simulink model "Katex_FullCar_R2017b_V03"  (R2026a)
settings: Solver=ode1  StopTime=1000  FixedStep=Ts  EnableMultiTasking=on
PostLoadFcn:
  | , if any(exist('dsrtsu_mdlpostloadfcn', 'file') == [2, 3, 6]), try dsrtsu_mdlpostloadfcn('Execute', bdroot); catch fprintf('Error in PostLoadFcn (dsrtsu_mdlpostloadfcn) for model "%s":\n %s\n', bdroot, lasterr); end, end,
  | , if any(exist('dsrtsu_mdlpostloadfcn', 'file') ~= 0), dsrtsu_mdlpostloadfcn('Execute', bdroot); end,
InitFcn:
  | , if any(exist('rtifpga_mdlclblib', 'file') ~= 0), rtifpga_mdlclblib('Init', bdroot); end,
  | 
  | 
  | init
undefined symbols (not defined in the file): locklim_sus, roundN, Ts
libraries: sl_discontinuities x29, simulink_extras x26, simulink x22, mjLib x1
(part 4 of 10)

== system Katex_FullCar_R2017b_V03/MuJoCo Interface/RR_Motor_Control/Drv_Driver ==
  In1 : Inport
  In2 : Inport  Port=2
  If1 : If  IfExpression=u1 == 0  ElseIfExpressions=u1 == 1,u1 == 2
  Merge : Merge  Inputs=3
  Position Mode : Subsystem  TreatAsAtomicUnit=on
  Torque Mode : Subsystem  TreatAsAtomicUnit=on
  Velocity Mode : Subsystem  TreatAsAtomicUnit=on
  RR_drive_motor : Outport
  wires:
  [wheel_radius] -> Velocity Mode/5(In5)
  [RRdrv_angvel_rads] -> Velocity Mode/4(In4)
  [drv_motor_freq] -> Velocity Mode/3(In3)
  [drv_motor_zeta] -> Velocity Mode/2(In2)
  Merge/1 -> RR_drive_motor/1
  In2/1 -> Position Mode/1(In1), Velocity Mode/1(In1), Torque Mode/1(In1)
  Velocity Mode/1(controlgain) -> Merge/2
  In1/1 -> If1/1
  Torque Mode/1(controlgain) -> Merge/3
  Position Mode/1(Out1) -> Merge/1
  If1/3 -> Torque Mode/Action
  If1/2 -> Velocity Mode/Action
  If1/1 -> Position Mode/Action

== system Katex_FullCar_R2017b_V03/MuJoCo Interface/RR_Motor_Control/Str_Driver ==
  In1 : Inport
  In2 : Inport  Port=2
  If1 : If  IfExpression=u1 == 0  ElseIfExpressions=u1 == 1,u1 == 2
  Merge : Merge  Inputs=3
  Position Mode : Subsystem  TreatAsAtomicUnit=on
  Torque Mode : Subsystem  TreatAsAtomicUnit=on
  Velocity Mode : Subsystem  TreatAsAtomicUnit=on
  RR_steer_motor : Outport
  wires:
  [RRstr_angvel_rads] -> Position Mode/5(velocity_rad_s)
  [RRstr_ang_rad] -> Position Mode/4(In4)
  [str_motor_freq] -> Position Mode/3(In3)
  [str_motor_zeta] -> Position Mode/2(In2)
  If1/1 -> Position Mode/Action
  If1/2 -> Velocity Mode/Action
  If1/3 -> Torque Mode/Action
  Position Mode/1(Out1) -> Merge/1
  Torque Mode/1(controlgain) -> Merge/3
  In1/1 -> If1/1
  Velocity Mode/1(Out1) -> Merge/2
  In2/1 -> Torque Mode/1(In1), Velocity Mode/1(In1), Position Mode/1(In1)
  Merge/1 -> RR_steer_motor/1

== system Katex_FullCar_R2017b_V03/MuJoCo Interface/RR_Motor_Control/Sus_Driver ==
  In1 : Inport
  In2 : Inport  Port=2
  If1 : If  IfExpression=u1 == 0  ElseIfExpressions=u1 == 1,u1 == 2
  Merge : Merge  Inputs=3
  Position Mode : Subsystem  TreatAsAtomicUnit=on
  Torque Mode : Subsystem  TreatAsAtomicUnit=on
  Velocity Mode : Subsystem  TreatAsAtomicUnit=on
  RR_sus_motor : Outport
  wires:
  [RRsus_angvel_rads] -> Position Mode/5(velocity_rad_s)
  [RRsus_ang_rad] -> Position Mode/4(In4)
  [sus_motor_freq] -> Position Mode/3(In3)
  [sus_motor_zeta] -> Position Mode/2(In2)
  Merge/1 -> RR_sus_motor/1
  In2/1 -> Velocity Mode/1(In1), Torque Mode/1(In1), Position Mode/1(In1)
  Velocity Mode/1(Out1) -> Merge/2
  In1/1 -> If1/1
  Torque Mode/1(controlgain) -> Merge/3
  Position Mode/1(Out1) -> Merge/1
  If1/3 -> Torque Mode/Action
  If1/2 -> Velocity Mode/Action
  If1/1 -> Position Mode/Action

== system Katex_FullCar_R2017b_V03/Scope/FL/Subsystem13 ==
  In1 : Inport
  Product : Product  Inputs=*/
  Out1 : Outport
  wires:
  In1/1 -> Product/1  "m/s"
  Product/1 -> Out1/1  "Load (rad/s)"
  [wheel_radius] -> Product/2

== system Katex_FullCar_R2017b_V03/DGIST/Attitude_reference_generator/Attitude Profile/LPF ==
  note: s = 2/Ts*(z-1)/(z+1)
  note: H(s) = 1/(tau*s+1)
  note: y(n) = [Ts*{x(n)+x(n-1)}+(2*tau-Ts)*y(n-1)]/(2*tau+Ts)
  note: LPF : tau = 1/(2*pi*fc)
  In : Inport
  fc : Inport  Port=2
  Constant : Constant  Value=Ts  SampleTime=Ts
  Constant1 : Constant  SampleTime=Ts
  Product1 : Product  Inputs=*/  RndMeth=Zero
  Product11 : Product  RndMeth=Zero
  Product2 : Product  Inputs=*/  RndMeth=Zero
  Sum1 : Sum  Inputs=+-  InputSameDT=on  SaturateOnIntegerOverflow=on  OutDataTypeStr=Inherit: Same as first input
  Sum2 : Sum  InputSameDT=on  SaturateOnIntegerOverflow=on  OutDataTypeStr=Inherit: Same as first input
  Sum3 : Sum  InputSameDT=on  SaturateOnIntegerOverflow=on  OutDataTypeStr=Inherit: Same as first input
  Sum4 : Sum  InputSameDT=on  SaturateOnIntegerOverflow=on  OutDataTypeStr=Inherit: Same as first input
  d : UnitDelay  SampleTime=Ts
  d1 : UnitDelay  SampleTime=Ts
  gain : Gain  Gain=Ts  SaturateOnIntegerOverflow=on  OutDataTypeStr=Inherit: Same as input  ParamDataTypeStr=Inherit: Same as input
  gain1 : Gain  Gain=2  SaturateOnIntegerOverflow=on  OutDataTypeStr=Inherit: Same as input  ParamDataTypeStr=Inherit: Same as input
  gain2 : Gain  Gain=2*pi  SaturateOnIntegerOverflow=on  OutDataTypeStr=Inherit: Same as input  ParamDataTypeStr=Inherit: Same as input
  Out : Outport  VectorParamsAs1DForOutWhenUnconnected=off
  wires:
  gain2/1 -> Product2/2
  Constant1/1 -> Product2/1
  Product2/1 -> gain1/1
  Product1/1 -> d/1, Out/1
  Sum4/1 -> Product1/2
  Sum2/1 -> Product1/1
  d/1 -> Product11/2
  gain1/1 -> Sum4/1, Sum1/1
  fc/1 -> gain2/1
  Constant/1 -> Sum4/2, Sum1/2
  Sum1/1 -> Product11/1
  Product11/1 -> Sum2/2
  gain/1 -> Sum2/1
  Sum3/1 -> gain/1
  d1/1 -> Sum3/2
  In/1 -> d1/1, Sum3/1

== system Katex_FullCar_R2017b_V03/DGIST/Attitude_reference_generator/Attitude Profile/LPF1 ==
  note: s = 2/Ts*(z-1)/(z+1)
  note: H(s) = 1/(tau*s+1)
  note: y(n) = [Ts*{x(n)+x(n-1)}+(2*tau-Ts)*y(n-1)]/(2*tau+Ts)
  note: LPF : tau = 1/(2*pi*fc)
  In : Inport
  fc : Inport  Port=2
  Constant : Constant  Value=Ts  SampleTime=Ts
  Constant1 : Constant  SampleTime=Ts
  Product1 : Product  Inputs=*/  RndMeth=Zero
  Product11 : Product  RndMeth=Zero
  Product2 : Product  Inputs=*/  RndMeth=Zero
  Sum1 : Sum  Inputs=+-  InputSameDT=on  SaturateOnIntegerOverflow=on  OutDataTypeStr=Inherit: Same as first input
  Sum2 : Sum  InputSameDT=on  SaturateOnIntegerOverflow=on  OutDataTypeStr=Inherit: Same as first input
  Sum3 : Sum  InputSameDT=on  SaturateOnIntegerOverflow=on  OutDataTypeStr=Inherit: Same as first input
  Sum4 : Sum  InputSameDT=on  SaturateOnIntegerOverflow=on  OutDataTypeStr=Inherit: Same as first input
  d : UnitDelay  SampleTime=Ts
  d1 : UnitDelay  SampleTime=Ts
  gain : Gain  Gain=Ts  SaturateOnIntegerOverflow=on  OutDataTypeStr=Inherit: Same as input  ParamDataTypeStr=Inherit: Same as input
  gain1 : Gain  Gain=2  SaturateOnIntegerOverflow=on  OutDataTypeStr=Inherit: Same as input  ParamDataTypeStr=Inherit: Same as input
  gain2 : Gain  Gain=2*pi  SaturateOnIntegerOverflow=on  OutDataTypeStr=Inherit: Same as input  ParamDataTypeStr=Inherit: Same as input
  Out : Outport  VectorParamsAs1DForOutWhenUnconnected=off
  wires:
  gain2/1 -> Product2/2
  Constant1/1 -> Product2/1
  Product2/1 -> gain1/1
  Product1/1 -> d/1, Out/1
  Sum4/1 -> Product1/2
  Sum2/1 -> Product1/1
  d/1 -> Product11/2
  gain1/1 -> Sum4/1, Sum1/1
  fc/1 -> gain2/1
  Constant/1 -> Sum4/2, Sum1/2
  Sum1/1 -> Product11/1
  Product11/1 -> Sum2/2
  gain/1 -> Sum2/1
  Sum3/1 -> gain/1
  d1/1 -> Sum3/2
  In/1 -> d1/1, Sum3/1

== system Katex_FullCar_R2017b_V03/DGIST/Attitude_reference_generator/Attitude Profile/LPF2 ==
  note: s = 2/Ts*(z-1)/(z+1)
  note: H(s) = 1/(tau*s+1)
  note: y(n) = [Ts*{x(n)+x(n-1)}+(2*tau-Ts)*y(n-1)]/(2*tau+Ts)
  note: LPF : tau = 1/(2*pi*fc)
  In : Inport
  fc : Inport  Port=2
  Constant : Constant  Value=Ts  SampleTime=Ts
  Constant1 : Constant  SampleTime=Ts
  Product1 : Product  Inputs=*/  RndMeth=Zero
  Product11 : Product  RndMeth=Zero
  Product2 : Product  Inputs=*/  RndMeth=Zero
  Sum1 : Sum  Inputs=+-  InputSameDT=on  SaturateOnIntegerOverflow=on  OutDataTypeStr=Inherit: Same as first input
  Sum2 : Sum  InputSameDT=on  SaturateOnIntegerOverflow=on  OutDataTypeStr=Inherit: Same as first input
  Sum3 : Sum  InputSameDT=on  SaturateOnIntegerOverflow=on  OutDataTypeStr=Inherit: Same as first input
  Sum4 : Sum  InputSameDT=on  SaturateOnIntegerOverflow=on  OutDataTypeStr=Inherit: Same as first input
  d : UnitDelay  SampleTime=Ts
  d1 : UnitDelay  SampleTime=Ts
  gain : Gain  Gain=Ts  SaturateOnIntegerOverflow=on  OutDataTypeStr=Inherit: Same as input  ParamDataTypeStr=Inherit: Same as input
  gain1 : Gain  Gain=2  SaturateOnIntegerOverflow=on  OutDataTypeStr=Inherit: Same as input  ParamDataTypeStr=Inherit: Same as input
  gain2 : Gain  Gain=2*pi  SaturateOnIntegerOverflow=on  OutDataTypeStr=Inherit: Same as input  ParamDataTypeStr=Inherit: Same as input
  Out : Outport  VectorParamsAs1DForOutWhenUnconnected=off
  wires:
  gain2/1 -> Product2/2
  Constant1/1 -> Product2/1
  Product2/1 -> gain1/1
  Product1/1 -> d/1, Out/1
  Sum4/1 -> Product1/2
  Sum2/1 -> Product1/1
  d/1 -> Product11/2
  gain1/1 -> Sum4/1, Sum1/1
  fc/1 -> gain2/1
  Constant/1 -> Sum4/2, Sum1/2
  Sum1/1 -> Product11/1
  Product11/1 -> Sum2/2
  gain/1 -> Sum2/1
  Sum3/1 -> gain/1
  d1/1 -> Sum3/2
  In/1 -> d1/1, Sum3/1

== system Katex_FullCar_R2017b_V03/DGIST/Attitude_reference_generator/Attitude Profile/LPF3 ==
  note: LPF : tau = 1/(2*pi*fc)
  note: y(n) = [Ts*{x(n)+x(n-1)}+(2*tau-Ts)*y(n-1)]/(2*tau+Ts)
  note: H(s) = 1/(tau*s+1)
  note: s = 2/Ts*(z-1)/(z+1)
  In : Inport
  fc : Inport  Port=2
  Constant : Constant  Value=Ts  SampleTime=Ts
  Constant1 : Constant  SampleTime=Ts
  Product1 : Product  Inputs=*/  RndMeth=Zero
  Product11 : Product  RndMeth=Zero
  Product2 : Product  Inputs=*/  RndMeth=Zero
  Sum1 : Sum  Inputs=+-  InputSameDT=on  SaturateOnIntegerOverflow=on  OutDataTypeStr=Inherit: Same as first input
  Sum2 : Sum  InputSameDT=on  SaturateOnIntegerOverflow=on  OutDataTypeStr=Inherit: Same as first input
  Sum3 : Sum  InputSameDT=on  SaturateOnIntegerOverflow=on  OutDataTypeStr=Inherit: Same as first input
  Sum4 : Sum  InputSameDT=on  SaturateOnIntegerOverflow=on  OutDataTypeStr=Inherit: Same as first input
  d : UnitDelay  SampleTime=Ts
  d1 : UnitDelay  SampleTime=Ts
  gain : Gain  Gain=Ts  SaturateOnIntegerOverflow=on  OutDataTypeStr=Inherit: Same as input  ParamDataTypeStr=Inherit: Same as input
  gain1 : Gain  Gain=2  SaturateOnIntegerOverflow=on  OutDataTypeStr=Inherit: Same as input  ParamDataTypeStr=Inherit: Same as input
  gain2 : Gain  Gain=2*pi  SaturateOnIntegerOverflow=on  OutDataTypeStr=Inherit: Same as input  ParamDataTypeStr=Inherit: Same as input
  Out : Outport  VectorParamsAs1DForOutWhenUnconnected=off
  wires:
  In/1 -> Sum3/1, d1/1
  d1/1 -> Sum3/2
  Sum3/1 -> gain/1
  gain/1 -> Sum2/1
  Product11/1 -> Sum2/2
  Sum1/1 -> Product11/1
  Constant/1 -> Sum1/2, Sum4/2
  fc/1 -> gain2/1
  gain1/1 -> Sum1/1, Sum4/1
  d/1 -> Product11/2
  Sum2/1 -> Product1/1
  Sum4/1 -> Product1/2
  Product1/1 -> Out/1, d/1
  Product2/1 -> gain1/1
  Constant1/1 -> Product2/1
  gain2/1 -> Product2/2

== system Katex_FullCar_R2017b_V03/DGIST/_High_Level_Ctrl/Chassis_FB_ctrl/P Control ==
  err : Inport
  Divide : Product  Inputs=**
  Out1 : Outport
  wires:
  err/1 -> Divide/1
  [Vx_FB_Kp] -> Divide/2
  Divide/1 -> Out1/1

== system Katex_FullCar_R2017b_V03/DGIST/_High_Level_Ctrl/Chassis_FB_ctrl/P Control1 ==
  err : Inport
  Divide : Product  Inputs=**
  Out1 : Outport
  wires:
  err/1 -> Divide/1
  [YawRate_FB_Kp] -> Divide/2
  Divide/1 -> Out1/1

== system Katex_FullCar_R2017b_V03/DGIST/_High_Level_Ctrl/Chassis_FB_ctrl/Slip contro FLl ==
  In1 : Inport
  Abs : Abs  SaturateOnIntegerOverflow=off
  Subsystem : Subsystem
  Switch : Switch  Criteria=u2 > Threshold  SaturateOnIntegerOverflow=off  InputSameDT=off
  Switch1 : Switch  Criteria=u2 > Threshold  Threshold=0.1  SaturateOnIntegerOverflow=off  InputSameDT=off
  Out1 : Outport  VectorParamsAs1DForOutWhenUnconnected=off
  wires:
  [Slip_Kp] -> Subsystem/3(Kgain)
  [Slip_Ctrl_OnOff] -> Switch/2
  Switch/1 -> Out1/1
  [Wheel_Radius] -> Subsystem/5(radius)
  [Avg_vel_meas] -> Subsystem/2(Dri_meas[m/s])
  [Slip_Limit] -> Subsystem/4(Slip Limit)
  Switch1/1 -> Switch/1
  In1/1 -> Abs/1, Switch1/3, Subsystem/1(Dri_ref[rad/s]), Switch/3
  Abs/1 -> Switch1/2
  Subsystem/1(omega*) -> Switch1/1

== system Katex_FullCar_R2017b_V03/DGIST/_High_Level_Ctrl/Chassis_FB_ctrl/Slip control FR ==
  In1 : Inport
  Abs : Abs  SaturateOnIntegerOverflow=off
  Subsystem : Subsystem
  Switch : Switch  Criteria=u2 > Threshold  SaturateOnIntegerOverflow=off  InputSameDT=off
  Switch1 : Switch  Criteria=u2 > Threshold  Threshold=0.1  SaturateOnIntegerOverflow=off  InputSameDT=off
  Out1 : Outport  VectorParamsAs1DForOutWhenUnconnected=off
  wires:
  Subsystem/1(omega*) -> Switch1/1
  Abs/1 -> Switch1/2
  In1/1 -> Switch/3, Subsystem/1(Dri_ref[rad/s]), Switch1/3, Abs/1
  Switch1/1 -> Switch/1
  [Slip_Limit] -> Subsystem/4(Slip Limit)
  [Avg_vel_meas] -> Subsystem/2(Dri_meas[m/s])
  [Wheel_Radius] -> Subsystem/5(radius)
  Switch/1 -> Out1/1
  [Slip_Ctrl_OnOff] -> Switch/2
  [Slip_Kp] -> Subsystem/3(Kgain)

== system Katex_FullCar_R2017b_V03/DGIST/_High_Level_Ctrl/Chassis_FB_ctrl/Subsystem3 ==
  In1 : Inport
  Constant2 : Constant
  Constant3 : Constant  Value=-1
  If : If  IfExpression=u1 >= 0  ElseIfExpressions=u1<0
  If Action Subsystem : Subsystem  TreatAsAtomicUnit=on
  If Action Subsystem1 : Subsystem  TreatAsAtomicUnit=on
  Merge : Merge
  sign : Outport  VectorParamsAs1DForOutWhenUnconnected=off
  wires:
  If/1 -> If Action Subsystem/Action
  If/2 -> If Action Subsystem1/Action
  Constant2/1 -> If Action Subsystem/1(In1)
  Merge/1 -> sign/1
  In1/1 -> If/1
  Constant3/1 -> If Action Subsystem1/1(In1)
  If Action Subsystem1/1(Out1) -> Merge/2
  If Action Subsystem/1(Out1) -> Merge/1

== system Katex_FullCar_R2017b_V03/DGIST/_High_Level_Ctrl/Chassis_FF_ctrl/P Control1 ==
  err : Inport
  Divide : Product  Inputs=**
  Out1 : Outport
  wires:
  err/1 -> Divide/1
  [YawRate_FB_Kp] -> Divide/2
  Divide/1 -> Out1/1

== system Katex_FullCar_R2017b_V03/DGIST/_High_Level_Ctrl/Orientation_Pos_Ctrl/Body_Pitch_PID_ctrl ==
  note: P Control
  In1 : Inport
  In2 : Inport  Port=2
  Add : Sum  Inputs=+-
  Add1 : Sum  Inputs=+-
  Divide1 : Product  Inputs=**
  Divide2 : Product  Inputs=**
  Out1 : Outport  VectorParamsAs1DForOutWhenUnconnected=off
  wires:
  Divide2/1 -> Add1/2
  Divide1/1 -> Divide2/1
  Add/1 -> Divide1/1
  [Pitch_Pos_Kp] -> Divide2/2
  Add1/1 -> Out1/1
  [Ori_Pos_PID_OnOff] -> Divide1/2
  In1/1 -> Add1/1, Add/1
  In2/1 -> Add/2

== system Katex_FullCar_R2017b_V03/DGIST/_High_Level_Ctrl/Orientation_Pos_Ctrl/Body_Roll_PID_ctrl ==
  note: P Control
  In1 : Inport
  In2 : Inport  Port=2
  Add : Sum  Inputs=+-
  Add1 : Sum  Inputs=+-
  Divide1 : Product  Inputs=**
  Divide2 : Product  Inputs=**
  Out1 : Outport  VectorParamsAs1DForOutWhenUnconnected=off
  wires:
  Divide2/1 -> Add1/2
  Divide1/1 -> Divide2/1
  Add/1 -> Divide1/1
  [Roll_Pos_Kp] -> Divide2/2
  Add1/1 -> Out1/1
  [Ori_Pos_PID_OnOff] -> Divide1/2
  In1/1 -> Add1/1, Add/1
  In2/1 -> Add/2

== system Katex_FullCar_R2017b_V03/DGIST/_Low_Level_Ctrl/Driving_Low_Level_Controller/FB Mode ==
  note: Load rad/s
  note: RPM
  note: Load m/s
  note: Load m/s
  In1 : Inport
  Action Port : ActionPort  ActionPortLabel=elseif(u1 == 3)
  Constant : Constant  Value=9
  Constant1 : Constant  Value=0
  Constant2 : Constant  Value=10
  Demux : Demux
  Dri_Loadradps_2_mps : Subsystem
      mask Display: disp('Dri_Loadradps_2_mps');
  Dri_Loadradps_2_mps1 : Subsystem
      mask Display: disp('Dri_Loadradps_2_mps');
  Mux : Mux
  Mux1 : Mux
  Out1 : Outport  VectorParamsAs1DForOutWhenUnconnected=off
  Out2 : Outport  Port=2  VectorParamsAs1DForOutWhenUnconnected=off
  wires:
  Mux/1 -> Out1/1
  Dri_Loadradps_2_mps/1(Out1) -> Mux/1
  Constant1/1 -> Mux/4, Mux/3
  Constant/1 -> Mux1/2, Mux1/1
  Mux1/1 -> Out2/1
  Dri_Loadradps_2_mps1/1(Out1) -> Mux/2
  Constant2/1 -> Mux1/4, Mux1/3
  In1/1 -> Demux/1
  Demux/1 -> Dri_Loadradps_2_mps/1(In1)
  Demux/2 -> Dri_Loadradps_2_mps1/1(In1)

== system Katex_FullCar_R2017b_V03/DGIST/_Low_Level_Ctrl/Driving_Low_Level_Controller/Torque Mode ==
  note: Load rad/s (Ref)
  note: Load rad/s (Measure)
  note: Target Torque
  note: Target Torque
  Action Port : ActionPort  ActionPortLabel=elseif(u1 == 2)
  Constant : Constant  Value=10
  Driving Wheel Control : Subsystem  Commented=on
      mask Display: disp('Driving Wheel Control')
  Mux : Mux
  Mux1 : Mux
  Out1 : Outport
  Out2 : Outport  Port=2
  wires:
  [DriRR_Load_Vel_Ref] -> ?
  [DriFL_Load_Vel_Ref] -> Driving Wheel Control/1(Ref)
  [DriRL_Load_Vel_Ref] -> ?
  [DriFR_Load_Vel_Ref] -> ?
  Driving Wheel Control/1(Target Torque) -> Mux/1
  ? -> Mux/2
  ? -> Mux/3
  ? -> Mux/4
  Mux/1 -> Out1/1
  Mux1/1 -> Out2/1
  Constant/1 -> Mux1/4, Mux1/3, Mux1/2, Mux1/1

== system Katex_FullCar_R2017b_V03/DGIST/_Low_Level_Ctrl/Driving_Low_Level_Controller/Tunning reference box ==
  Constant1 : Constant  Value=0
  Gain1 : Gain
  Mux1 : Mux
  Sine Wave1 : Sin  Amplitude=10  Frequency=0.2  SampleTime=0
  Out1 : Outport
  Out2 : Outport  Port=2
  wires:
  Mux1/1 -> Out2/1
  Sine Wave1/1 -> Gain1/1
  Gain1/1 -> Mux1/2, Mux1/3, Mux1/4, Mux1/1
  Constant1/1 -> Out1/1

== system Katex_FullCar_R2017b_V03/DGIST/_Low_Level_Ctrl/Driving_Low_Level_Controller/Velocity Mode ==
  note: Load rad/s
  note: Load m/s
  note: Load m/s
  In1 : Inport
  Action Port : ActionPort  ActionPortLabel=if(u1 == 1)
  Constant : Constant  Value=9
  Demux : Demux
  Dri_Loadradps_2_mps : Subsystem
      mask Display: disp('Dri_Loadradps_2_mps');
  Dri_Loadradps_2_mps1 : Subsystem
      mask Display: disp('Dri_Loadradps_2_mps');
  Dri_Loadradps_2_mps2 : Subsystem
      mask Display: disp('Dri_Loadradps_2_mps');
  Dri_Loadradps_2_mps3 : Subsystem
      mask Display: disp('Dri_Loadradps_2_mps');
  Mux : Mux
  Mux1 : Mux
  Out1 : Outport  VectorParamsAs1DForOutWhenUnconnected=off
  Out2 : Outport  Port=2  VectorParamsAs1DForOutWhenUnconnected=off
  wires:
  Dri_Loadradps_2_mps/1(Out1) -> Mux/1
  Dri_Loadradps_2_mps2/1(Out1) -> Mux/3
  Dri_Loadradps_2_mps3/1(Out1) -> Mux/4
  Constant/1 -> Mux1/4, Mux1/3, Mux1/2, Mux1/1
  Mux1/1 -> Out2/1
  Dri_Loadradps_2_mps1/1(Out1) -> Mux/2
  In1/1 -> Demux/1
  Demux/1 -> Dri_Loadradps_2_mps/1(In1)
  Demux/2 -> Dri_Loadradps_2_mps1/1(In1)
  Demux/3 -> Dri_Loadradps_2_mps2/1(In1)
  Demux/4 -> Dri_Loadradps_2_mps3/1(In1)
  Mux/1 -> Out1/1

== system Katex_FullCar_R2017b_V03/DGIST/_Low_Level_Ctrl/Steering_Low_Level_Controller/Position Mode ==
  note: Load deg
  note: Load deg
  note: Load deg
  note: Load deg
  note: Load deg
  In1 : Inport
  Action Port : ActionPort  ActionPortLabel=if(u1 == 0)
  Constant : Constant  Value=8
  Demux : Demux
  Mux : Mux
  Mux1 : Mux
  Out1 : Outport  VectorParamsAs1DForOutWhenUnconnected=off
  Out2 : Outport  Port=2  VectorParamsAs1DForOutWhenUnconnected=off
  wires:
  Mux/1 -> Out1/1
  Constant/1 -> Mux1/4, Mux1/3, Mux1/2, Mux1/1
  Mux1/1 -> Out2/1
  In1/1 -> Demux/1
  Demux/1 -> Mux/1
  Demux/2 -> Mux/2
  Demux/3 -> Mux/3
  Demux/4 -> Mux/4

== system Katex_FullCar_R2017b_V03/DGIST/_Low_Level_Ctrl/Steering_Low_Level_Controller/Torque Mode ==
  note: DOB check 필요
  note: Load deg
  note: Motor Target Torque
  note: Load deg (Measure)
  Action Port : ActionPort  ActionPortLabel=elseif(u1 == 2)
  Constant : Constant  Value=10
  Mux : Mux
  Mux1 : Mux
  Steering Motor Control : Subsystem  Commented=on
      mask Display: disp('Steering Motor Control')
  Steering Motor Control1 : Subsystem  Commented=on
      mask Display: disp('Steering Motor Control')
  Steering Motor Control2 : Subsystem  Commented=on
      mask Display: disp('Steering Motor Control')
  Steering Motor Control3 : Subsystem  Commented=on
      mask Display: disp('Steering Motor Control')
  Out1 : Outport  VectorParamsAs1DForOutWhenUnconnected=off
  Out2 : Outport  Port=2  VectorParamsAs1DForOutWhenUnconnected=off
  wires:
  Mux/1 -> Out1/1
  Constant/1 -> Mux1/4, Mux1/3, Mux1/2, Mux1/1
  Mux1/1 -> Out2/1
  Steering Motor Control/1(Out1) -> Mux/1
  [StrFL_Load_Pos_Ref] -> Steering Motor Control/1(In1)
  [StrFR_Load_Pos_Ref] -> Steering Motor Control1/1(In1)
  Steering Motor Control1/1(Out1) -> Mux/2
  Steering Motor Control2/1(Out1) -> Mux/3
  [StrRL_Load_Pos_Ref] -> Steering Motor Control2/1(In1)
  Steering Motor Control3/1(Out1) -> Mux/4
  [StrRR_Load_Pos_Ref] -> Steering Motor Control3/1(In1)

== system Katex_FullCar_R2017b_V03/DGIST/_Low_Level_Ctrl/Suspension_Low_Level_Controller/Position Mode ==
  note: Load deg
  note: Load deg
  In1 : Inport
  In2 : Inport  Port=2
  Action Port : ActionPort  ActionPortLabel=if(u1 == 0)
  Constant : Constant  Value=8
  Demux : Demux
  Gain{,1..3} (4 alike) : Gain  Gain=-1
  Mux : Mux
  Mux1 : Mux
  Saturation Dynamic{,1..3} (4 alike) : sl_discontinuities/Saturation Dynamic  OutMin=[]  OutMax=[]  OutDataTypeStr=Inherit: Same as second input  OutDataType=fixdt(1, 16)  OutScaling=2^-10  DoSatur=off
  Out1 : Outport  VectorParamsAs1DForOutWhenUnconnected=off
  Out2 : Outport  Port=2  VectorParamsAs1DForOutWhenUnconnected=off
  wires:
  Mux/1 -> Out1/1
  Constant/1 -> Mux1/4, Mux1/3, Mux1/2, Mux1/1
  Mux1/1 -> Out2/1
  Demux/1 -> Saturation Dynamic/2
  Saturation Dynamic/1 -> Mux/1
  Saturation Dynamic1/1 -> Mux/2
  Demux/2 -> Saturation Dynamic1/2
  Demux/3 -> Saturation Dynamic2/2
  Saturation Dynamic2/1 -> Mux/3
  Demux/4 -> Saturation Dynamic3/2
  Saturation Dynamic3/1 -> Mux/4
  Gain/1 -> Saturation Dynamic/3
  Gain1/1 -> Saturation Dynamic1/3
  Gain2/1 -> Saturation Dynamic2/3
  In2/1 -> Gain3/1, Saturation Dynamic3/1, Gain2/1, Saturation Dynamic2/1, Gain1/1, Saturation Dynamic1/1, Gain/1, Saturation Dynamic/1
  Gain3/1 -> Saturation Dynamic3/3
  In1/1 -> Demux/1

== system Katex_FullCar_R2017b_V03/DGIST/_Low_Level_Ctrl/Suspension_Low_Level_Controller/Torque Mode ==
  note: Target Torque
  In1 : Inport
  In2 : Inport  Port=2
  Action Port : ActionPort  ActionPortLabel=elseif(u1 == 2)
  Constant : Constant  Value=10
  Demux : Demux
  Gain{,1..3} (4 alike) : Gain  Gain=-1
  Mux : Mux
  Mux1 : Mux
  Saturation Dynamic{,1..3} (4 alike) : sl_discontinuities/Saturation Dynamic  OutMin=[]  OutMax=[]  OutDataTypeStr=Inherit: Same as second input  OutDataType=fixdt(1, 16)  OutScaling=2^-10  DoSatur=off
  Subsystem : Subsystem  Commented=on
      mask Display: disp('Suspension Motor Control')
  Out1 : Outport
  Out2 : Outport  Port=2
  wires:
  Mux1/1 -> Out2/1
  Constant/1 -> Mux1/4, Mux1/3, Mux1/2, Mux1/1
  Gain/1 -> Saturation Dynamic/3
  Saturation Dynamic1/1 -> Mux/2
  Gain2/1 -> Saturation Dynamic2/3
  Demux/4 -> Saturation Dynamic3/2
  In2/1 -> Gain3/1, Saturation Dynamic3/1, Gain2/1, Saturation Dynamic2/1, Gain1/1, Saturation Dynamic1/1, Gain/1, Saturation Dynamic/1
  Saturation Dynamic3/1 -> Mux/4
  Demux/3 -> Saturation Dynamic2/2
  Demux/2 -> Saturation Dynamic1/2
  Demux/1 -> Saturation Dynamic/2
  Gain3/1 -> Saturation Dynamic3/3
  Gain1/1 -> Saturation Dynamic1/3
  Saturation Dynamic2/1 -> Mux/3
  Saturation Dynamic/1 -> Mux/1
  In1/1 -> Demux/1
  Mux/1 -> Out1/1

== system Katex_FullCar_R2017b_V03/DGIST/_Low_Level_Ctrl/Suspension_Low_Level_Controller/Tunning reference box ==
  Constant1 : Constant  Value=0
  Gain1 : Gain
  Mux1 : Mux
  Mux2 : Mux
  Sine Wave1 : Sin  Amplitude=10  Frequency=0.2  SampleTime=0
  Out1 : Outport
  Out2 : Outport  Port=2
  wires:
  Mux1/1 -> Out2/1
  Sine Wave1/1 -> Gain1/1
  Gain1/1 -> Mux1/2, Mux1/3, Mux1/4, Mux1/1
  Constant1/1 -> Mux2/4, Mux2/3, Mux2/2, Mux2/1
  Mux2/1 -> Out1/1

== system Katex_FullCar_R2017b_V03/DGIST/_Low_Level_Ctrl/Suspension_Low_Level_Controller/Velocity Mode ==
  note: Load rad/s
  note: RPM
  note: RPM
  Action Port : ActionPort  ActionPortLabel=elseif(u1 == 1)
  Constant : Constant  Value=9
  Mux : Mux
  Mux1 : Mux
  Sus_LoadVel_2_MotorRPM : Subsystem  Commented=on
      mask Display: disp('Sus_LoadVel_2_MotorRPM');
  Sus_LoadVel_2_MotorRPM1 : Subsystem  Commented=on
      mask Display: disp('Sus_LoadVel_2_MotorRPM');
  Sus_LoadVel_2_MotorRPM2 : Subsystem  Commented=on
      mask Display: disp('Sus_LoadVel_2_MotorRPM');
  Sus_LoadVel_2_MotorRPM3 : Subsystem  Commented=on
      mask Display: disp('Sus_LoadVel_2_MotorRPM');
  Out1 : Outport  VectorParamsAs1DForOutWhenUnconnected=off
  Out2 : Outport  Port=2  VectorParamsAs1DForOutWhenUnconnected=off
  wires:
  Mux/1 -> Out1/1
  [SusFL_Load_Vel_Ref] -> Sus_LoadVel_2_MotorRPM/1(In1)
  [SusFR_Load_Vel_Ref] -> Sus_LoadVel_2_MotorRPM1/1(In1)
  [SusRL_Load_Vel_Ref] -> Sus_LoadVel_2_MotorRPM2/1(In1)
  [SusRR_Load_Vel_Ref] -> Sus_LoadVel_2_MotorRPM3/1(In1)
  Sus_LoadVel_2_MotorRPM/1(Out1) -> Mux/1
  Sus_LoadVel_2_MotorRPM2/1(Out1) -> Mux/3
  Sus_LoadVel_2_MotorRPM3/1(Out1) -> Mux/4
  Constant/1 -> Mux1/4, Mux1/3, Mux1/2, Mux1/1
  Mux1/1 -> Out2/1
  Sus_LoadVel_2_MotorRPM1/1(Out1) -> Mux/2

== system Katex_FullCar_R2017b_V03/DGIST/_Reference_Generator/Slalom Profile/LPF ==
  note: LPF : tau = 1/(2*pi*fc)
  note: y(n) = [Ts*{x(n)+x(n-1)}+(2*tau-Ts)*y(n-1)]/(2*tau+Ts)
  note: H(s) = 1/(tau*s+1)
  note: s = 2/Ts*(z-1)/(z+1)
  In : Inport
  fc : Inport  Port=2
  Constant : Constant  Value=Ts  SampleTime=Ts
  Constant1 : Constant  SampleTime=Ts
  Product1 : Product  Inputs=*/  RndMeth=Zero
  Product11 : Product  RndMeth=Zero
  Product2 : Product  Inputs=*/  RndMeth=Zero
  Sum1 : Sum  Inputs=+-  InputSameDT=on  SaturateOnIntegerOverflow=on  OutDataTypeStr=Inherit: Same as first input
  Sum2 : Sum  InputSameDT=on  SaturateOnIntegerOverflow=on  OutDataTypeStr=Inherit: Same as first input
  Sum3 : Sum  InputSameDT=on  SaturateOnIntegerOverflow=on  OutDataTypeStr=Inherit: Same as first input
  Sum4 : Sum  InputSameDT=on  SaturateOnIntegerOverflow=on  OutDataTypeStr=Inherit: Same as first input
  d : UnitDelay  SampleTime=Ts
  d1 : UnitDelay  SampleTime=Ts
  gain : Gain  Gain=Ts  SaturateOnIntegerOverflow=on  OutDataTypeStr=Inherit: Same as input  ParamDataTypeStr=Inherit: Same as input
  gain1 : Gain  Gain=2  SaturateOnIntegerOverflow=on  OutDataTypeStr=Inherit: Same as input  ParamDataTypeStr=Inherit: Same as input
  gain2 : Gain  Gain=2*pi  SaturateOnIntegerOverflow=on  OutDataTypeStr=Inherit: Same as input  ParamDataTypeStr=Inherit: Same as input
  Out : Outport  VectorParamsAs1DForOutWhenUnconnected=off
  wires:
  In/1 -> Sum3/1, d1/1
  d1/1 -> Sum3/2
  Sum3/1 -> gain/1
  gain/1 -> Sum2/1
  Product11/1 -> Sum2/2
  Sum1/1 -> Product11/1
  Constant/1 -> Sum1/2, Sum4/2
  fc/1 -> gain2/1
  gain1/1 -> Sum1/1, Sum4/1
  d/1 -> Product11/2
  Sum2/1 -> Product1/1
  Sum4/1 -> Product1/2
  Product1/1 -> Out/1, d/1
  Product2/1 -> gain1/1
  Constant1/1 -> Product2/1
  gain2/1 -> Product2/2

== system Katex_FullCar_R2017b_V03/DGIST/_Reference_Generator/Slalom Profile/LPF1 ==
  note: LPF : tau = 1/(2*pi*fc)
  note: y(n) = [Ts*{x(n)+x(n-1)}+(2*tau-Ts)*y(n-1)]/(2*tau+Ts)
  note: H(s) = 1/(tau*s+1)
  note: s = 2/Ts*(z-1)/(z+1)
  In : Inport
  fc : Inport  Port=2
  Constant : Constant  Value=Ts  SampleTime=Ts
  Constant1 : Constant  SampleTime=Ts
  Product1 : Product  Inputs=*/  RndMeth=Zero
  Product11 : Product  RndMeth=Zero
  Product2 : Product  Inputs=*/  RndMeth=Zero
  Sum1 : Sum  Inputs=+-  InputSameDT=on  SaturateOnIntegerOverflow=on  OutDataTypeStr=Inherit: Same as first input
  Sum2 : Sum  InputSameDT=on  SaturateOnIntegerOverflow=on  OutDataTypeStr=Inherit: Same as first input
  Sum3 : Sum  InputSameDT=on  SaturateOnIntegerOverflow=on  OutDataTypeStr=Inherit: Same as first input
  Sum4 : Sum  InputSameDT=on  SaturateOnIntegerOverflow=on  OutDataTypeStr=Inherit: Same as first input
  d : UnitDelay  SampleTime=Ts
  d1 : UnitDelay  SampleTime=Ts
  gain : Gain  Gain=Ts  SaturateOnIntegerOverflow=on  OutDataTypeStr=Inherit: Same as input  ParamDataTypeStr=Inherit: Same as input
  gain1 : Gain  Gain=2  SaturateOnIntegerOverflow=on  OutDataTypeStr=Inherit: Same as input  ParamDataTypeStr=Inherit: Same as input
  gain2 : Gain  Gain=2*pi  SaturateOnIntegerOverflow=on  OutDataTypeStr=Inherit: Same as input  ParamDataTypeStr=Inherit: Same as input
  Out : Outport  VectorParamsAs1DForOutWhenUnconnected=off
  wires:
  In/1 -> Sum3/1, d1/1
  d1/1 -> Sum3/2
  Sum3/1 -> gain/1
  gain/1 -> Sum2/1
  Product11/1 -> Sum2/2
  Sum1/1 -> Product11/1
  Constant/1 -> Sum1/2, Sum4/2
  fc/1 -> gain2/1
  gain1/1 -> Sum1/1, Sum4/1
  d/1 -> Product11/2
  Sum2/1 -> Product1/1
  Sum4/1 -> Product1/2
  Product1/1 -> Out/1, d/1
  Product2/1 -> gain1/1
  Constant1/1 -> Product2/1
  gain2/1 -> Product2/2

== system Katex_FullCar_R2017b_V03/DGIST/_Reference_Generator/Slalom Profile/LPF2 ==
  note: LPF : tau = 1/(2*pi*fc)
  note: y(n) = [Ts*{x(n)+x(n-1)}+(2*tau-Ts)*y(n-1)]/(2*tau+Ts)
  note: H(s) = 1/(tau*s+1)
  note: s = 2/Ts*(z-1)/(z+1)
  In : Inport
  fc : Inport  Port=2
  Constant : Constant  Value=Ts  SampleTime=Ts
  Constant1 : Constant  SampleTime=Ts
  Product1 : Product  Inputs=*/  RndMeth=Zero
  Product11 : Product  RndMeth=Zero
  Product2 : Product  Inputs=*/  RndMeth=Zero
  Sum1 : Sum  Inputs=+-  InputSameDT=on  SaturateOnIntegerOverflow=on  OutDataTypeStr=Inherit: Same as first input
  Sum2 : Sum  InputSameDT=on  SaturateOnIntegerOverflow=on  OutDataTypeStr=Inherit: Same as first input
  Sum3 : Sum  InputSameDT=on  SaturateOnIntegerOverflow=on  OutDataTypeStr=Inherit: Same as first input
  Sum4 : Sum  InputSameDT=on  SaturateOnIntegerOverflow=on  OutDataTypeStr=Inherit: Same as first input
  d : UnitDelay  SampleTime=Ts
  d1 : UnitDelay  SampleTime=Ts
  gain : Gain  Gain=Ts  SaturateOnIntegerOverflow=on  OutDataTypeStr=Inherit: Same as input  ParamDataTypeStr=Inherit: Same as input
  gain1 : Gain  Gain=2  SaturateOnIntegerOverflow=on  OutDataTypeStr=Inherit: Same as input  ParamDataTypeStr=Inherit: Same as input
  gain2 : Gain  Gain=2*pi  SaturateOnIntegerOverflow=on  OutDataTypeStr=Inherit: Same as input  ParamDataTypeStr=Inherit: Same as input
  Out : Outport  VectorParamsAs1DForOutWhenUnconnected=off
  wires:
  In/1 -> Sum3/1, d1/1
  d1/1 -> Sum3/2
  Sum3/1 -> gain/1
  gain/1 -> Sum2/1
  Product11/1 -> Sum2/2
  Sum1/1 -> Product11/1
  Constant/1 -> Sum1/2, Sum4/2
  fc/1 -> gain2/1
  gain1/1 -> Sum1/1, Sum4/1
  d/1 -> Product11/2
  Sum2/1 -> Product1/1
  Sum4/1 -> Product1/2
  Product1/1 -> Out/1, d/1
  Product2/1 -> gain1/1
  Constant1/1 -> Product2/1
  gain2/1 -> Product2/2

== system Katex_FullCar_R2017b_V03/DGIST/_Reference_Generator/Straight Profile/LPF ==
  note: LPF : tau = 1/(2*pi*fc)
  note: y(n) = [Ts*{x(n)+x(n-1)}+(2*tau-Ts)*y(n-1)]/(2*tau+Ts)
  note: H(s) = 1/(tau*s+1)
  note: s = 2/Ts*(z-1)/(z+1)
  In : Inport
  fc : Inport  Port=2
  Constant : Constant  Value=Ts  SampleTime=Ts
  Constant1 : Constant  SampleTime=Ts
  Product1 : Product  Inputs=*/  RndMeth=Zero
  Product11 : Product  RndMeth=Zero
  Product2 : Product  Inputs=*/  RndMeth=Zero
  Sum1 : Sum  Inputs=+-  InputSameDT=on  SaturateOnIntegerOverflow=on  OutDataTypeStr=Inherit: Same as first input
  Sum2 : Sum  InputSameDT=on  SaturateOnIntegerOverflow=on  OutDataTypeStr=Inherit: Same as first input
  Sum3 : Sum  InputSameDT=on  SaturateOnIntegerOverflow=on  OutDataTypeStr=Inherit: Same as first input
  Sum4 : Sum  InputSameDT=on  SaturateOnIntegerOverflow=on  OutDataTypeStr=Inherit: Same as first input
  d : UnitDelay  SampleTime=Ts
  d1 : UnitDelay  SampleTime=Ts
  gain : Gain  Gain=Ts  SaturateOnIntegerOverflow=on  OutDataTypeStr=Inherit: Same as input  ParamDataTypeStr=Inherit: Same as input
  gain1 : Gain  Gain=2  SaturateOnIntegerOverflow=on  OutDataTypeStr=Inherit: Same as input  ParamDataTypeStr=Inherit: Same as input
  gain2 : Gain  Gain=2*pi  SaturateOnIntegerOverflow=on  OutDataTypeStr=Inherit: Same as input  ParamDataTypeStr=Inherit: Same as input
  Out : Outport  VectorParamsAs1DForOutWhenUnconnected=off
  wires:
  In/1 -> Sum3/1, d1/1
  d1/1 -> Sum3/2
  Sum3/1 -> gain/1
  gain/1 -> Sum2/1
  Product11/1 -> Sum2/2
  Sum1/1 -> Product11/1
  Constant/1 -> Sum1/2, Sum4/2
  fc/1 -> gain2/1
  gain1/1 -> Sum1/1, Sum4/1
  d/1 -> Product11/2
  Sum2/1 -> Product1/1
  Sum4/1 -> Product1/2
  Product1/1 -> Out/1, d/1
  Product2/1 -> gain1/1
  Constant1/1 -> Product2/1
  gain2/1 -> Product2/2

== system Katex_FullCar_R2017b_V03/DGIST/_Reference_Generator/Straight Profile/LPF1 ==
  note: LPF : tau = 1/(2*pi*fc)
  note: y(n) = [Ts*{x(n)+x(n-1)}+(2*tau-Ts)*y(n-1)]/(2*tau+Ts)
  note: H(s) = 1/(tau*s+1)
  note: s = 2/Ts*(z-1)/(z+1)
  In : Inport
  fc : Inport  Port=2
  Constant : Constant  Value=Ts  SampleTime=Ts
  Constant1 : Constant  SampleTime=Ts
  Product1 : Product  Inputs=*/  RndMeth=Zero
  Product11 : Product  RndMeth=Zero
  Product2 : Product  Inputs=*/  RndMeth=Zero
  Sum1 : Sum  Inputs=+-  InputSameDT=on  SaturateOnIntegerOverflow=on  OutDataTypeStr=Inherit: Same as first input
  Sum2 : Sum  InputSameDT=on  SaturateOnIntegerOverflow=on  OutDataTypeStr=Inherit: Same as first input
  Sum3 : Sum  InputSameDT=on  SaturateOnIntegerOverflow=on  OutDataTypeStr=Inherit: Same as first input
  Sum4 : Sum  InputSameDT=on  SaturateOnIntegerOverflow=on  OutDataTypeStr=Inherit: Same as first input
  d : UnitDelay  SampleTime=Ts
  d1 : UnitDelay  SampleTime=Ts
  gain : Gain  Gain=Ts  SaturateOnIntegerOverflow=on  OutDataTypeStr=Inherit: Same as input  ParamDataTypeStr=Inherit: Same as input
  gain1 : Gain  Gain=2  SaturateOnIntegerOverflow=on  OutDataTypeStr=Inherit: Same as input  ParamDataTypeStr=Inherit: Same as input
  gain2 : Gain  Gain=2*pi  SaturateOnIntegerOverflow=on  OutDataTypeStr=Inherit: Same as input  ParamDataTypeStr=Inherit: Same as input
  Out : Outport  VectorParamsAs1DForOutWhenUnconnected=off
  wires:
  In/1 -> Sum3/1, d1/1
  d1/1 -> Sum3/2
  Sum3/1 -> gain/1
  gain/1 -> Sum2/1
  Product11/1 -> Sum2/2
  Sum1/1 -> Product11/1
  Constant/1 -> Sum1/2, Sum4/2
  fc/1 -> gain2/1
  gain1/1 -> Sum1/1, Sum4/1
  d/1 -> Product11/2
  Sum2/1 -> Product1/1
  Sum4/1 -> Product1/2
  Product1/1 -> Out/1, d/1
  Product2/1 -> gain1/1
  Constant1/1 -> Product2/1
  gain2/1 -> Product2/2

== system Katex_FullCar_R2017b_V03/DGIST/_Reference_Generator/Straight Profile/LPF2 ==
  note: LPF : tau = 1/(2*pi*fc)
  note: y(n) = [Ts*{x(n)+x(n-1)}+(2*tau-Ts)*y(n-1)]/(2*tau+Ts)
  note: H(s) = 1/(tau*s+1)
  note: s = 2/Ts*(z-1)/(z+1)
  In : Inport
  fc : Inport  Port=2
  Constant : Constant  Value=Ts  SampleTime=Ts
  Constant1 : Constant  SampleTime=Ts
  Product1 : Product  Inputs=*/  RndMeth=Zero
  Product11 : Product  RndMeth=Zero
  Product2 : Product  Inputs=*/  RndMeth=Zero
  Sum1 : Sum  Inputs=+-  InputSameDT=on  SaturateOnIntegerOverflow=on  OutDataTypeStr=Inherit: Same as first input
  Sum2 : Sum  InputSameDT=on  SaturateOnIntegerOverflow=on  OutDataTypeStr=Inherit: Same as first input
  Sum3 : Sum  InputSameDT=on  SaturateOnIntegerOverflow=on  OutDataTypeStr=Inherit: Same as first input
  Sum4 : Sum  InputSameDT=on  SaturateOnIntegerOverflow=on  OutDataTypeStr=Inherit: Same as first input
  d : UnitDelay  SampleTime=Ts
  d1 : UnitDelay  SampleTime=Ts
  gain : Gain  Gain=Ts  SaturateOnIntegerOverflow=on  OutDataTypeStr=Inherit: Same as input  ParamDataTypeStr=Inherit: Same as input
  gain1 : Gain  Gain=2  SaturateOnIntegerOverflow=on  OutDataTypeStr=Inherit: Same as input  ParamDataTypeStr=Inherit: Same as input
  gain2 : Gain  Gain=2*pi  SaturateOnIntegerOverflow=on  OutDataTypeStr=Inherit: Same as input  ParamDataTypeStr=Inherit: Same as input
  Out : Outport  VectorParamsAs1DForOutWhenUnconnected=off
  wires:
  In/1 -> Sum3/1, d1/1
  d1/1 -> Sum3/2
  Sum3/1 -> gain/1
  gain/1 -> Sum2/1
  Product11/1 -> Sum2/2
  Sum1/1 -> Product11/1
  Constant/1 -> Sum1/2, Sum4/2
  fc/1 -> gain2/1
  gain1/1 -> Sum1/1, Sum4/1
  d/1 -> Product11/2
  Sum2/1 -> Product1/1
  Sum4/1 -> Product1/2
  Product1/1 -> Out/1, d/1
  Product2/1 -> gain1/1
  Constant1/1 -> Product2/1
  gain2/1 -> Product2/2

== system Katex_FullCar_R2017b_V03/Locomotion/Conditioning/Steering mode/If Action Subsystem ==
  Action Port : ActionPort  ActionPortLabel=if(u1==1)
  Mux : Mux
  Mux1 : Mux
  offsetFL : Constant  Value=0
  offsetFR : Constant  Value=0
  offsetRL : Constant  Value=0
  offsetRR : Constant  Value=0
  signFL : Constant
  signFR : Constant
  signRL : Constant  Value=0
  signRR : Constant  Value=0
  sign : Outport  VectorParamsAs1DForOutWhenUnconnected=off
  offset : Outport  Port=2  VectorParamsAs1DForOutWhenUnconnected=off
  wires:
  Mux/1 -> sign/1
  signFL/1 -> Mux/1  "signFL"
  signFR/1 -> Mux/2  "signFR"
  signRL/1 -> Mux/3  "signRL"
  signRR/1 -> Mux/4  "signRR"
  offsetRR/1 -> Mux1/4  "offsetRR"
  offsetRL/1 -> Mux1/3  "offsetRL"
  offsetFR/1 -> Mux1/2  "offsetFR"
  offsetFL/1 -> Mux1/1  "offsetFL"
  Mux1/1 -> offset/1

== system Katex_FullCar_R2017b_V03/Locomotion/Conditioning/Steering mode/If Action Subsystem1 ==
  Action Port : ActionPort  ActionPortLabel=elseif(u1==2)
  Mux : Mux
  Mux1 : Mux
  offsetFL : Constant  Value=0
  offsetFR : Constant  Value=0
  offsetRL : Constant  Value=0
  offsetRR : Constant  Value=0
  signFL : Constant
  signFR : Constant
  signRL : Constant
  signRR : Constant
  sign : Outport  VectorParamsAs1DForOutWhenUnconnected=off
  offset : Outport  Port=2  VectorParamsAs1DForOutWhenUnconnected=off
  wires:
  signRR/1 -> Mux/4  "signRR"
  signRL/1 -> Mux/3  "signRL"
  signFR/1 -> Mux/2  "signFR"
  signFL/1 -> Mux/1  "signFL"
  Mux/1 -> sign/1
  offsetFR/1 -> Mux1/2  "offsetFR"
  offsetFL/1 -> Mux1/1  "offsetFL"
  Mux1/1 -> offset/1
  offsetRR/1 -> Mux1/4  "offsetRR"
  offsetRL/1 -> Mux1/3  "offsetRL"

== system Katex_FullCar_R2017b_V03/Locomotion/Conditioning/Steering mode/If Action Subsystem2 ==
  Action Port : ActionPort  ActionPortLabel=elseif(u1==3)
  Mux : Mux
  Mux1 : Mux
  offsetFL : Constant  Value=0
  offsetFR : Constant  Value=0
  offsetRL : Constant  Value=0
  offsetRR : Constant  Value=0
  signFL : Constant
  signFR : Constant
  signRL : Constant  Value=-1
  signRR : Constant  Value=-1
  sign : Outport  VectorParamsAs1DForOutWhenUnconnected=off
  offset : Outport  Port=2  VectorParamsAs1DForOutWhenUnconnected=off
  wires:
  Mux/1 -> sign/1
  signFL/1 -> Mux/1  "signFL"
  signFR/1 -> Mux/2  "signFR"
  signRL/1 -> Mux/3  "signRL"
  signRR/1 -> Mux/4  "signRR"
  offsetRL/1 -> Mux1/3  "offsetRL"
  offsetRR/1 -> Mux1/4  "offsetRR"
  Mux1/1 -> offset/1
  offsetFL/1 -> Mux1/1  "offsetFL"
  offsetFR/1 -> Mux1/2  "offsetFR"

== system Katex_FullCar_R2017b_V03/Locomotion/Conditioning/Steering mode/If Action Subsystem3 ==
  In1 : Inport
  Action Port : ActionPort  ActionPortLabel=elseif(u1==4)
  Multiply : Product
  Mux : Mux
  Mux1 : Mux
  offsetFL : Constant  Value=-43.43
  offsetFR : Constant  Value=43.43
  offsetRL : Constant  Value=43.43
  offsetRR : Constant  Value=-43.43
  signFL : Constant  Value=0
  signFR : Constant  Value=0
  signRL : Constant  Value=0
  signRR : Constant  Value=0
  sign : Outport  VectorParamsAs1DForOutWhenUnconnected=off
  offset : Outport  Port=2  VectorParamsAs1DForOutWhenUnconnected=off
  wires:
  signRR/1 -> Mux/4  "signRR"
  signRL/1 -> Mux/3  "signRL"
  signFR/1 -> Mux/2  "signFR"
  signFL/1 -> Mux/1  "signFL"
  Mux/1 -> sign/1
  offsetRL/1 -> Mux1/3  "offsetRL"
  offsetRR/1 -> Mux1/4  "offsetRR"
  Mux1/1 -> Multiply/1
  offsetFL/1 -> Mux1/1  "offsetFL"
  offsetFR/1 -> Mux1/2  "offsetFR"
  In1/1 -> Multiply/2
  Multiply/1 -> offset/1

== system Katex_FullCar_R2017b_V03/Locomotion/Conditioning/Suspension mode/If Action Subsystem ==
  Action Port : ActionPort  ActionPortLabel=if(u1==0)
  Mux : Mux
  enableFL : Constant
  enableFR : Constant
  enableRL : Constant
  enableRR : Constant
  enable : Outport  VectorParamsAs1DForOutWhenUnconnected=off
  wires:
  Mux/1 -> enable/1
  enableFL/1 -> Mux/1  "enableFL"
  enableFR/1 -> Mux/2  "enableFR"
  enableRL/1 -> Mux/3  "enableRL"
  enableRR/1 -> Mux/4  "enableRR"

== system Katex_FullCar_R2017b_V03/Locomotion/Conditioning/Suspension mode/If Action Subsystem1 ==
  Action Port : ActionPort  ActionPortLabel=elseif(u1==1)
  Mux : Mux
  enableFL : Constant
  enableFR : Constant  Value=0
  enableRL : Constant  Value=0
  enableRR : Constant  Value=0
  enable : Outport  VectorParamsAs1DForOutWhenUnconnected=off
  wires:
  enableRR/1 -> Mux/4  "enableRR"
  enableRL/1 -> Mux/3  "enableRL"
  enableFR/1 -> Mux/2  "enableFR"
  enableFL/1 -> Mux/1  "enableFL"
  Mux/1 -> enable/1

== system Katex_FullCar_R2017b_V03/Locomotion/Conditioning/Suspension mode/If Action Subsystem2 ==
  Action Port : ActionPort  ActionPortLabel=elseif(u1==2)
  Mux : Mux
  enableFL : Constant  Value=0
  enableFR : Constant
  enableRL : Constant  Value=0
  enableRR : Constant  Value=0
  enable : Outport  VectorParamsAs1DForOutWhenUnconnected=off
  wires:
  Mux/1 -> enable/1
  enableFL/1 -> Mux/1  "enableFL"
  enableFR/1 -> Mux/2  "enableFR"
  enableRL/1 -> Mux/3  "enableRL"
  enableRR/1 -> Mux/4  "enableRR"

== system Katex_FullCar_R2017b_V03/Locomotion/Conditioning/Suspension mode/If Action Subsystem3 ==
  Action Port : ActionPort  ActionPortLabel=elseif(u1==3)
  Mux : Mux
  enableFL : Constant  Value=0
  enableFR : Constant  Value=0
  enableRL : Constant
  enableRR : Constant  Value=0
  enable : Outport  VectorParamsAs1DForOutWhenUnconnected=off
  wires:
  enableRR/1 -> Mux/4  "enableRR"
  enableRL/1 -> Mux/3  "enableRL"
  enableFR/1 -> Mux/2  "enableFR"
  enableFL/1 -> Mux/1  "enableFL"
  Mux/1 -> enable/1

== system Katex_FullCar_R2017b_V03/Locomotion/Conditioning/Suspension mode/If Action Subsystem4 ==
  Action Port : ActionPort  ActionPortLabel=elseif(u1==4)
  Mux : Mux
  enableFL : Constant  Value=0
  enableFR : Constant  Value=0
  enableRL : Constant  Value=0
  enableRR : Constant
  enable : Outport  VectorParamsAs1DForOutWhenUnconnected=off
  wires:
  Mux/1 -> enable/1
  enableFL/1 -> Mux/1  "enableFL"
  enableFR/1 -> Mux/2  "enableFR"
  enableRL/1 -> Mux/3  "enableRL"
  enableRR/1 -> Mux/4  "enableRR"

== system Katex_FullCar_R2017b_V03/MuJoCo Interface/FL_Motor_Control/Drv_Driver/Position Mode ==
  In1 : Inport
  Action Port : ActionPort  ActionPortLabel=if(u1 == 0)
  Constant : Constant  Value=0
  Terminator : Terminator
  Out1 : Outport  VectorParamsAs1DForOutWhenUnconnected=off
  wires:
  Constant/1 -> Out1/1
  In1/1 -> Terminator/1

== system Katex_FullCar_R2017b_V03/MuJoCo Interface/FL_Motor_Control/Drv_Driver/Torque Mode ==
  In1 : Inport
  Action Port : ActionPort  ActionPortLabel=elseif(u1 == 2)
  Bus Selector1 : BusSelector  OutputSignals=FL_tqctrl.FLdrv_tqref_pct
  controlgain : Outport  VectorParamsAs1DForOutWhenUnconnected=off
  wires:
  Bus Selector1/1 -> controlgain/1  "<FLdrv_tqref_pct>"
  In1/1 -> Bus Selector1/1

== system Katex_FullCar_R2017b_V03/MuJoCo Interface/FL_Motor_Control/Drv_Driver/Velocity Mode ==
  In1 : Inport
  In2 : Inport  Port=2
  In3 : Inport  Port=3
  In4 : Inport  Port=4
  In5 : Inport  Port=5
  Action Port : ActionPort  ActionPortLabel=elseif(u1 == 1)
  Bus Selector1 : BusSelector  OutputSignals=FLdrv_velref_mps
  FL_vel_velocity_motor_driver : Subsystem
  Subsystem13 : Subsystem
      mask Display: disp('Dri_ref(m/s)_2_motor(rad/s)');
  controlgain : Outport  VectorParamsAs1DForOutWhenUnconnected=off
  wires:
  In1/1 -> Bus Selector1/1
  FL_vel_velocity_motor_driver/1(controlgain) -> controlgain/1
  Bus Selector1/1 -> Subsystem13/1(In1)  "<FLdrv_velref_mps>"
  Subsystem13/1(Out1) -> FL_vel_velocity_motor_driver/1(In1)
  In2/1 -> FL_vel_velocity_motor_driver/2(In2)
  In3/1 -> FL_vel_velocity_motor_driver/3(In3)
  In4/1 -> FL_vel_velocity_motor_driver/4(In4)
  In5/1 -> Subsystem13/2(In2)

== system Katex_FullCar_R2017b_V03/MuJoCo Interface/FL_Motor_Control/Str_Driver/Position Mode ==
  In1 : Inport
  In2 : Inport  Port=2
  In3 : Inport  Port=3
  In4 : Inport  Port=4
  velocity_rad_s : Inport  Port=5
  Action Port : ActionPort  ActionPortLabel=if(u1 == 0)
  Bus Selector1 : BusSelector  OutputSignals=FLstr_angref_deg
  Degrees to Radians1 : simulink_extras/Transformations/Degrees to Radians
  FL_str_position_motor_driver : Subsystem
  Out1 : Outport  VectorParamsAs1DForOutWhenUnconnected=off
  wires:
  In1/1 -> Bus Selector1/1
  Degrees to Radians1/1 -> FL_str_position_motor_driver/1(In1)
  Bus Selector1/1 -> Degrees to Radians1/1  "<FLstr_angref_deg>"
  FL_str_position_motor_driver/1(Out1) -> Out1/1
  In2/1 -> FL_str_position_motor_driver/2(In2)
  In3/1 -> FL_str_position_motor_driver/3(In3)
  In4/1 -> FL_str_position_motor_driver/4(In4)
  velocity_rad_s/1 -> FL_str_position_motor_driver/5(velocity_rad_s)

== system Katex_FullCar_R2017b_V03/MuJoCo Interface/FL_Motor_Control/Str_Driver/Torque Mode ==
  In1 : Inport
  Action Port : ActionPort  ActionPortLabel=elseif(u1 == 2)
  Bus Selector1 : BusSelector  OutputSignals=FL_tqctrl.FLstr_tqref_pct
  controlgain : Outport  VectorParamsAs1DForOutWhenUnconnected=off
  wires:
  In1/1 -> Bus Selector1/1
  Bus Selector1/1 -> controlgain/1  "<FLstr_tqref_pct>"

== system Katex_FullCar_R2017b_V03/MuJoCo Interface/FL_Motor_Control/Str_Driver/Velocity Mode ==
  In1 : Inport
  Action Port : ActionPort  ActionPortLabel=elseif(u1 == 1)
  Constant : Constant  Value=0
  Terminator : Terminator
  Out1 : Outport  VectorParamsAs1DForOutWhenUnconnected=off
  wires:
  Constant/1 -> Out1/1
  In1/1 -> Terminator/1

== system Katex_FullCar_R2017b_V03/MuJoCo Interface/FL_Motor_Control/Sus_Driver/Position Mode ==
  In1 : Inport
  In2 : Inport  Port=2
  In3 : Inport  Port=3
  In4 : Inport  Port=4
  velocity_rad_s : Inport  Port=5
  Action Port : ActionPort  ActionPortLabel=if(u1 == 0)
  Bus Selector : BusSelector  OutputSignals=FLsus_angref_deg
  Degrees to Radians : simulink_extras/Transformations/Degrees to Radians
  FL_sus_position_motor_driver : Subsystem
  Out1 : Outport  VectorParamsAs1DForOutWhenUnconnected=off
  wires:
  Degrees to Radians/1 -> FL_sus_position_motor_driver/1(In1)
  FL_sus_position_motor_driver/1(Out1) -> Out1/1
  In1/1 -> Bus Selector/1
  Bus Selector/1 -> Degrees to Radians/1  "<FLsus_angref_deg>"
  In2/1 -> FL_sus_position_motor_driver/2(In2)
  In3/1 -> FL_sus_position_motor_driver/3(In3)
  In4/1 -> FL_sus_position_motor_driver/4(In4)
  velocity_rad_s/1 -> FL_sus_position_motor_driver/5(velocity_rad_s)

== system Katex_FullCar_R2017b_V03/MuJoCo Interface/FL_Motor_Control/Sus_Driver/Torque Mode ==
  In1 : Inport
  Action Port : ActionPort  ActionPortLabel=elseif(u1 == 2)
  Bus Selector1 : BusSelector  OutputSignals=FL_tqctrl.FLsus_tqref_pct
  Scope : Scope
      settings: ActiveDisplayYMinimum=-1  ActiveDisplayYMaximum=1  DataLoggingVariableName=ScopeData78
  controlgain : Outport  VectorParamsAs1DForOutWhenUnconnected=off
  wires:
  Bus Selector1/1 -> Scope/1, controlgain/1  "<FLsus_tqref_pct>"
  In1/1 -> Bus Selector1/1

== system Katex_FullCar_R2017b_V03/MuJoCo Interface/FL_Motor_Control/Sus_Driver/Velocity Mode ==
  In1 : Inport
  Action Port : ActionPort  ActionPortLabel=elseif(u1 == 1)
  Constant : Constant  Value=0
  Terminator : Terminator
  Out1 : Outport  VectorParamsAs1DForOutWhenUnconnected=off
  wires:
  Constant/1 -> Out1/1
  In1/1 -> Terminator/1

== system Katex_FullCar_R2017b_V03/MuJoCo Interface/FR_Motor_Control/Drv_Driver/Position Mode ==
  In1 : Inport
  Action Port : ActionPort  ActionPortLabel=if(u1 == 0)
  Constant : Constant  Value=0
  Terminator : Terminator
  Out1 : Outport  VectorParamsAs1DForOutWhenUnconnected=off
  wires:
  In1/1 -> Terminator/1
  Constant/1 -> Out1/1

== system Katex_FullCar_R2017b_V03/MuJoCo Interface/FR_Motor_Control/Drv_Driver/Torque Mode ==
  In1 : Inport
  Action Port : ActionPort  ActionPortLabel=elseif(u1 == 2)
  Bus Selector1 : BusSelector  OutputSignals=FR_tqctrl.FRdrv_tqref_pct
  controlgain : Outport  VectorParamsAs1DForOutWhenUnconnected=off
  wires:
  In1/1 -> Bus Selector1/1
  Bus Selector1/1 -> controlgain/1  "<FRdrv_tqref_pct>"

== system Katex_FullCar_R2017b_V03/MuJoCo Interface/FR_Motor_Control/Drv_Driver/Velocity Mode ==
  In1 : Inport
  In2 : Inport  Port=2
  In3 : Inport  Port=3
  In4 : Inport  Port=4
  In5 : Inport  Port=5
  Action Port : ActionPort  ActionPortLabel=elseif(u1 == 1)
  Bus Selector1 : BusSelector  OutputSignals=FRdrv_velref_mps
  FR_vel_velocity_motor_driver : Subsystem
  Subsystem13 : Subsystem
      mask Display: disp('Dri_ref(m/s)_2_motor(rad/s)');
  controlgain : Outport  VectorParamsAs1DForOutWhenUnconnected=off
  wires:
  In5/1 -> Subsystem13/2(In2)
  In4/1 -> FR_vel_velocity_motor_driver/4(In4)
  In3/1 -> FR_vel_velocity_motor_driver/3(In3)
  In2/1 -> FR_vel_velocity_motor_driver/2(In2)
  Subsystem13/1(Out1) -> FR_vel_velocity_motor_driver/1(In1)
  Bus Selector1/1 -> Subsystem13/1(In1)  "<FRdrv_velref_mps>"
  FR_vel_velocity_motor_driver/1(controlgain) -> controlgain/1
  In1/1 -> Bus Selector1/1

== system Katex_FullCar_R2017b_V03/MuJoCo Interface/FR_Motor_Control/Str_Driver/Position Mode ==
  In1 : Inport
  In2 : Inport  Port=2
  In3 : Inport  Port=3
  In4 : Inport  Port=4
  velocity_rad_s : Inport  Port=5
  Action Port : ActionPort  ActionPortLabel=if(u1 == 0)
  Bus Selector1 : BusSelector  OutputSignals=FRstr_angref_deg
  Degrees to Radians1 : simulink_extras/Transformations/Degrees to Radians
  FR_str_position_motor_driver : Subsystem
  Out1 : Outport  VectorParamsAs1DForOutWhenUnconnected=off
  wires:
  velocity_rad_s/1 -> FR_str_position_motor_driver/5(velocity_rad_s)
  In4/1 -> FR_str_position_motor_driver/4(In4)
  In3/1 -> FR_str_position_motor_driver/3(In3)
  In2/1 -> FR_str_position_motor_driver/2(In2)
  FR_str_position_motor_driver/1(Out1) -> Out1/1
  Bus Selector1/1 -> Degrees to Radians1/1  "<FRstr_angref_deg>"
  Degrees to Radians1/1 -> FR_str_position_motor_driver/1(In1)
  In1/1 -> Bus Selector1/1

== system Katex_FullCar_R2017b_V03/MuJoCo Interface/FR_Motor_Control/Str_Driver/Torque Mode ==
  In1 : Inport
  Action Port : ActionPort  ActionPortLabel=elseif(u1 == 2)
  Bus Selector1 : BusSelector  OutputSignals=FR_tqctrl.FRstr_tqref_pct
  controlgain : Outport  VectorParamsAs1DForOutWhenUnconnected=off
  wires:
  Bus Selector1/1 -> controlgain/1  "<FRstr_tqref_pct>"
  In1/1 -> Bus Selector1/1
